simulink model "gm_hybrid_lht"  (R2019b)
settings: Solver=FixedStepDiscrete  StartTime=0.0  StopTime=inf  FixedStep=1/120e6  RelTol=1e-3
undefined symbols (not defined in the file or in its folder): bt, height, nTheta, width
libraries: hdlsllib x352, simulink x286, hdlmdlgenlib x7, dspsrcs4 x1
(part 9 of 12)

== system gm_hybrid_lht/Hybrid LHT/Hybrid LHT Accumulator/Accumulator with Switches/Accumulator_instance33/Block RAM/Simple Dual Port RAM Generator ==
  wr_data : Inport  OutDataTypeStr=fixdt(0, 36, 0)  PortDimensions=1  SampleTime=8.33333333333333e-09
  wr_addr : Inport  Port=2  OutDataTypeStr=fixdt(0, 11, 0)  PortDimensions=1  SampleTime=8.33333333333333e-09
  wr_en : Inport  Port=3  OutDataTypeStr=boolean  PortDimensions=1  SampleTime=8.33333333333333e-09
  rd_addr : Inport  Port=4  OutDataTypeStr=fixdt(0, 11, 0)  PortDimensions=1  SampleTime=8.33333333333333e-09
  and_0 : Logic  AllPortsSameDT=off  OutDataTypeStr=boolean
  and_1 : Logic  AllPortsSameDT=off  OutDataTypeStr=boolean
  bitwise_or : simulink/Logic and Bit Operations/Bitwise Operator  logicop=OR  UseBitMask=off  BitMask=bin2dec('11011001')  BitMaskRealWorld=Stored Integer
  constant_0 : Constant  Value=0  OutDataTypeStr=fixdt(0, 2, 0)  SampleTime=-1
  constant_1 : Constant  OutDataTypeStr=fixdt(0, 2, 0)  SampleTime=-1
  delay : Delay  DelayLength=1
  multiport_switch : MultiPortSwitch  DataPortOrder=Zero-based contiguous  Inputs=2  zeroidx=on
  rd_address : hdlsllib/Logic and Bit Operations/Bit Slice  lidx=9  ridx=0
      settings: SourceProductName=Simulink  SourceProductBaseCode=SL
  rd_address_hr : hdlsllib/Logic and Bit Operations/Bit Slice  lidx=8  ridx=0
      settings: SourceProductName=Simulink  SourceProductBaseCode=SL
  rd_bitslice : hdlsllib/Logic and Bit Operations/Bit Slice  lidx=10  ridx=10
      settings: SourceProductName=Simulink  SourceProductBaseCode=SL
  rd_cmp2const_0 : simulink/Logic and Bit Operations/Compare To Constant  relop===  const=0  OutDataTypeStr=boolean
  rd_cmp2const_1 : simulink/Logic and Bit Operations/Compare To Constant  relop===  const=1  OutDataTypeStr=boolean
  simple_ram_0 : hdlsllib/HDL RAMs/Simple Dual Port RAM  ram_size=10
      settings: SourceProductName=Simulink  SourceProductBaseCode=SL
  simple_ram_1 : hdlsllib/HDL RAMs/Simple Dual Port RAM  ram_size=9
      settings: SourceProductName=Simulink  SourceProductBaseCode=SL
  switch_0 : Switch  Threshold=1
  switch_1 : Switch  Threshold=1
  vector_concatenate : Concatenate
  wr_address : hdlsllib/Logic and Bit Operations/Bit Slice  lidx=9  ridx=0
      settings: SourceProductName=Simulink  SourceProductBaseCode=SL
  wr_address_hr : hdlsllib/Logic and Bit Operations/Bit Slice  lidx=8  ridx=0
      settings: SourceProductName=Simulink  SourceProductBaseCode=SL
  wr_bitslice : hdlsllib/Logic and Bit Operations/Bit Slice  lidx=10  ridx=10
      settings: SourceProductName=Simulink  SourceProductBaseCode=SL
  wr_cmp2const_0 : simulink/Logic and Bit Operations/Compare To Constant  relop===  const=0  OutDataTypeStr=boolean
  wr_cmp2const_1 : simulink/Logic and Bit Operations/Compare To Constant  relop===  const=1  OutDataTypeStr=boolean
  zero : Constant  Value=0  OutDataTypeStr=fixdt(0, 2, 0)  SampleTime=-1
  rd_data : Outport
  wires:
  rd_addr/1 -> rd_bitslice/1, rd_address_hr/1, rd_address/1
  wr_en/1 -> and_1/2, and_0/2
  wr_addr/1 -> wr_bitslice/1, wr_address_hr/1, wr_address/1
  wr_data/1 -> simple_ram_0/1, simple_ram_1/1
  and_0/1 -> simple_ram_0/3
  and_1/1 -> simple_ram_1/3
  bitwise_or/1 -> delay/1
  constant_0/1 -> switch_0/1
  constant_1/1 -> switch_1/1
  delay/1 -> multiport_switch/1
  multiport_switch/1 -> rd_data/1
  rd_address/1 -> simple_ram_0/4
  rd_address_hr/1 -> simple_ram_1/4
  rd_bitslice/1 -> rd_cmp2const_1/1, rd_cmp2const_0/1
  rd_cmp2const_0/1 -> switch_0/2
  rd_cmp2const_1/1 -> switch_1/2
  simple_ram_0/1 -> multiport_switch/2
  simple_ram_1/1 -> multiport_switch/3
  switch_0/1 -> vector_concatenate/1
  switch_1/1 -> vector_concatenate/2
  vector_concatenate/1 -> bitwise_or/1
  wr_address/1 -> simple_ram_0/2
  wr_address_hr/1 -> simple_ram_1/2
  wr_bitslice/1 -> wr_cmp2const_1/1, wr_cmp2const_0/1
  wr_cmp2const_0/1 -> and_0/1
  wr_cmp2const_1/1 -> and_1/1
  zero/1 -> switch_1/3, switch_0/3

== system gm_hybrid_lht/Hybrid LHT/Hybrid LHT Accumulator/Accumulator with Switches/Accumulator_instance34/Block RAM/Simple Dual Port RAM Generator ==
  wr_data : Inport  OutDataTypeStr=fixdt(0, 36, 0)  PortDimensions=1  SampleTime=8.33333333333333e-09
  wr_addr : Inport  Port=2  OutDataTypeStr=fixdt(0, 11, 0)  PortDimensions=1  SampleTime=8.33333333333333e-09
  wr_en : Inport  Port=3  OutDataTypeStr=boolean  PortDimensions=1  SampleTime=8.33333333333333e-09
  rd_addr : Inport  Port=4  OutDataTypeStr=fixdt(0, 11, 0)  PortDimensions=1  SampleTime=8.33333333333333e-09
  and_0 : Logic  AllPortsSameDT=off  OutDataTypeStr=boolean
  and_1 : Logic  AllPortsSameDT=off  OutDataTypeStr=boolean
  bitwise_or : simulink/Logic and Bit Operations/Bitwise Operator  logicop=OR  UseBitMask=off  BitMask=bin2dec('11011001')  BitMaskRealWorld=Stored Integer
  constant_0 : Constant  Value=0  OutDataTypeStr=fixdt(0, 2, 0)  SampleTime=-1
  constant_1 : Constant  OutDataTypeStr=fixdt(0, 2, 0)  SampleTime=-1
  delay : Delay  DelayLength=1
  multiport_switch : MultiPortSwitch  DataPortOrder=Zero-based contiguous  Inputs=2  zeroidx=on
  rd_address : hdlsllib/Logic and Bit Operations/Bit Slice  lidx=9  ridx=0
      settings: SourceProductName=Simulink  SourceProductBaseCode=SL
  rd_address_hr : hdlsllib/Logic and Bit Operations/Bit Slice  lidx=8  ridx=0
      settings: SourceProductName=Simulink  SourceProductBaseCode=SL
  rd_bitslice : hdlsllib/Logic and Bit Operations/Bit Slice  lidx=10  ridx=10
      settings: SourceProductName=Simulink  SourceProductBaseCode=SL
  rd_cmp2const_0 : simulink/Logic and Bit Operations/Compare To Constant  relop===  const=0  OutDataTypeStr=boolean
  rd_cmp2const_1 : simulink/Logic and Bit Operations/Compare To Constant  relop===  const=1  OutDataTypeStr=boolean
  simple_ram_0 : hdlsllib/HDL RAMs/Simple Dual Port RAM  ram_size=10
      settings: SourceProductName=Simulink  SourceProductBaseCode=SL
  simple_ram_1 : hdlsllib/HDL RAMs/Simple Dual Port RAM  ram_size=9
      settings: SourceProductName=Simulink  SourceProductBaseCode=SL
  switch_0 : Switch  Threshold=1
  switch_1 : Switch  Threshold=1
  vector_concatenate : Concatenate
  wr_address : hdlsllib/Logic and Bit Operations/Bit Slice  lidx=9  ridx=0
      settings: SourceProductName=Simulink  SourceProductBaseCode=SL
  wr_address_hr : hdlsllib/Logic and Bit Operations/Bit Slice  lidx=8  ridx=0
      settings: SourceProductName=Simulink  SourceProductBaseCode=SL
  wr_bitslice : hdlsllib/Logic and Bit Operations/Bit Slice  lidx=10  ridx=10
      settings: SourceProductName=Simulink  SourceProductBaseCode=SL
  wr_cmp2const_0 : simulink/Logic and Bit Operations/Compare To Constant  relop===  const=0  OutDataTypeStr=boolean
  wr_cmp2const_1 : simulink/Logic and Bit Operations/Compare To Constant  relop===  const=1  OutDataTypeStr=boolean
  zero : Constant  Value=0  OutDataTypeStr=fixdt(0, 2, 0)  SampleTime=-1
  rd_data : Outport
  wires:
  rd_addr/1 -> rd_bitslice/1, rd_address_hr/1, rd_address/1
  wr_en/1 -> and_1/2, and_0/2
  wr_addr/1 -> wr_bitslice/1, wr_address_hr/1, wr_address/1
  wr_data/1 -> simple_ram_0/1, simple_ram_1/1
  and_0/1 -> simple_ram_0/3
  and_1/1 -> simple_ram_1/3
  bitwise_or/1 -> delay/1
  constant_0/1 -> switch_0/1
  constant_1/1 -> switch_1/1
  delay/1 -> multiport_switch/1
  multiport_switch/1 -> rd_data/1
  rd_address/1 -> simple_ram_0/4
  rd_address_hr/1 -> simple_ram_1/4
  rd_bitslice/1 -> rd_cmp2const_1/1, rd_cmp2const_0/1
  rd_cmp2const_0/1 -> switch_0/2
  rd_cmp2const_1/1 -> switch_1/2
  simple_ram_0/1 -> multiport_switch/2
  simple_ram_1/1 -> multiport_switch/3
  switch_0/1 -> vector_concatenate/1
  switch_1/1 -> vector_concatenate/2
  vector_concatenate/1 -> bitwise_or/1
  wr_address/1 -> simple_ram_0/2
  wr_address_hr/1 -> simple_ram_1/2
  wr_bitslice/1 -> wr_cmp2const_1/1, wr_cmp2const_0/1
  wr_cmp2const_0/1 -> and_0/1
  wr_cmp2const_1/1 -> and_1/1
  zero/1 -> switch_1/3, switch_0/3

== system gm_hybrid_lht/Hybrid LHT/Hybrid LHT Accumulator/Accumulator with Switches/Accumulator_instance4/Block RAM/Simple Dual Port RAM Generator ==
  wr_data : Inport  OutDataTypeStr=fixdt(0, 36, 0)  PortDimensions=1  SampleTime=8.33333333333333e-09
  wr_addr : Inport  Port=2  OutDataTypeStr=fixdt(0, 11, 0)  PortDimensions=1  SampleTime=8.33333333333333e-09
  wr_en : Inport  Port=3  OutDataTypeStr=boolean  PortDimensions=1  SampleTime=8.33333333333333e-09
  rd_addr : Inport  Port=4  OutDataTypeStr=fixdt(0, 11, 0)  PortDimensions=1  SampleTime=8.33333333333333e-09
  and_0 : Logic  AllPortsSameDT=off  OutDataTypeStr=boolean
  and_1 : Logic  AllPortsSameDT=off  OutDataTypeStr=boolean
  bitwise_or : simulink/Logic and Bit Operations/Bitwise Operator  logicop=OR  UseBitMask=off  BitMask=bin2dec('11011001')  BitMaskRealWorld=Stored Integer
  constant_0 : Constant  Value=0  OutDataTypeStr=fixdt(0, 2, 0)  SampleTime=-1
  constant_1 : Constant  OutDataTypeStr=fixdt(0, 2, 0)  SampleTime=-1
  delay : Delay  DelayLength=1
  multiport_switch : MultiPortSwitch  DataPortOrder=Zero-based contiguous  Inputs=2  zeroidx=on
  rd_address : hdlsllib/Logic and Bit Operations/Bit Slice  lidx=9  ridx=0
      settings: SourceProductName=Simulink  SourceProductBaseCode=SL
  rd_address_hr : hdlsllib/Logic and Bit Operations/Bit Slice  lidx=8  ridx=0
      settings: SourceProductName=Simulink  SourceProductBaseCode=SL
  rd_bitslice : hdlsllib/Logic and Bit Operations/Bit Slice  lidx=10  ridx=10
      settings: SourceProductName=Simulink  SourceProductBaseCode=SL
  rd_cmp2const_0 : simulink/Logic and Bit Operations/Compare To Constant  relop===  const=0  OutDataTypeStr=boolean
  rd_cmp2const_1 : simulink/Logic and Bit Operations/Compare To Constant  relop===  const=1  OutDataTypeStr=boolean
  simple_ram_0 : hdlsllib/HDL RAMs/Simple Dual Port RAM  ram_size=10
      settings: SourceProductName=Simulink  SourceProductBaseCode=SL
  simple_ram_1 : hdlsllib/HDL RAMs/Simple Dual Port RAM  ram_size=9
      settings: SourceProductName=Simulink  SourceProductBaseCode=SL
  switch_0 : Switch  Threshold=1
  switch_1 : Switch  Threshold=1
  vector_concatenate : Concatenate
  wr_address : hdlsllib/Logic and Bit Operations/Bit Slice  lidx=9  ridx=0
      settings: SourceProductName=Simulink  SourceProductBaseCode=SL
  wr_address_hr : hdlsllib/Logic and Bit Operations/Bit Slice  lidx=8  ridx=0
      settings: SourceProductName=Simulink  SourceProductBaseCode=SL
  wr_bitslice : hdlsllib/Logic and Bit Operations/Bit Slice  lidx=10  ridx=10
      settings: SourceProductName=Simulink  SourceProductBaseCode=SL
  wr_cmp2const_0 : simulink/Logic and Bit Operations/Compare To Constant  relop===  const=0  OutDataTypeStr=boolean
  wr_cmp2const_1 : simulink/Logic and Bit Operations/Compare To Constant  relop===  const=1  OutDataTypeStr=boolean
  zero : Constant  Value=0  OutDataTypeStr=fixdt(0, 2, 0)  SampleTime=-1
  rd_data : Outport
  wires:
  rd_addr/1 -> rd_bitslice/1, rd_address_hr/1, rd_address/1
  wr_en/1 -> and_1/2, and_0/2
  wr_addr/1 -> wr_bitslice/1, wr_address_hr/1, wr_address/1
  wr_data/1 -> simple_ram_0/1, simple_ram_1/1
  and_0/1 -> simple_ram_0/3
  and_1/1 -> simple_ram_1/3
  bitwise_or/1 -> delay/1
  constant_0/1 -> switch_0/1
  constant_1/1 -> switch_1/1
  delay/1 -> multiport_switch/1
  multiport_switch/1 -> rd_data/1
  rd_address/1 -> simple_ram_0/4
  rd_address_hr/1 -> simple_ram_1/4
  rd_bitslice/1 -> rd_cmp2const_1/1, rd_cmp2const_0/1
  rd_cmp2const_0/1 -> switch_0/2
  rd_cmp2const_1/1 -> switch_1/2
  simple_ram_0/1 -> multiport_switch/2
  simple_ram_1/1 -> multiport_switch/3
  switch_0/1 -> vector_concatenate/1
  switch_1/1 -> vector_concatenate/2
  vector_concatenate/1 -> bitwise_or/1
  wr_address/1 -> simple_ram_0/2
  wr_address_hr/1 -> simple_ram_1/2
  wr_bitslice/1 -> wr_cmp2const_1/1, wr_cmp2const_0/1
  wr_cmp2const_0/1 -> and_0/1
  wr_cmp2const_1/1 -> and_1/1
  zero/1 -> switch_1/3, switch_0/3

== system gm_hybrid_lht/Hybrid LHT/Hybrid LHT Accumulator/Accumulator with Switches/Accumulator_instance5/Block RAM/Simple Dual Port RAM Generator ==
  wr_data : Inport  OutDataTypeStr=fixdt(0, 36, 0)  PortDimensions=1  SampleTime=8.33333333333333e-09
  wr_addr : Inport  Port=2  OutDataTypeStr=fixdt(0, 11, 0)  PortDimensions=1  SampleTime=8.33333333333333e-09
  wr_en : Inport  Port=3  OutDataTypeStr=boolean  PortDimensions=1  SampleTime=8.33333333333333e-09
  rd_addr : Inport  Port=4  OutDataTypeStr=fixdt(0, 11, 0)  PortDimensions=1  SampleTime=8.33333333333333e-09
  and_0 : Logic  AllPortsSameDT=off  OutDataTypeStr=boolean
  and_1 : Logic  AllPortsSameDT=off  OutDataTypeStr=boolean
  bitwise_or : simulink/Logic and Bit Operations/Bitwise Operator  logicop=OR  UseBitMask=off  BitMask=bin2dec('11011001')  BitMaskRealWorld=Stored Integer
  constant_0 : Constant  Value=0  OutDataTypeStr=fixdt(0, 2, 0)  SampleTime=-1
  constant_1 : Constant  OutDataTypeStr=fixdt(0, 2, 0)  SampleTime=-1
  delay : Delay  DelayLength=1
  multiport_switch : MultiPortSwitch  DataPortOrder=Zero-based contiguous  Inputs=2  zeroidx=on
  rd_address : hdlsllib/Logic and Bit Operations/Bit Slice  lidx=9  ridx=0
      settings: SourceProductName=Simulink  SourceProductBaseCode=SL
  rd_address_hr : hdlsllib/Logic and Bit Operations/Bit Slice  lidx=8  ridx=0
      settings: SourceProductName=Simulink  SourceProductBaseCode=SL
  rd_bitslice : hdlsllib/Logic and Bit Operations/Bit Slice  lidx=10  ridx=10
      settings: SourceProductName=Simulink  SourceProductBaseCode=SL
  rd_cmp2const_0 : simulink/Logic and Bit Operations/Compare To Constant  relop===  const=0  OutDataTypeStr=boolean
  rd_cmp2const_1 : simulink/Logic and Bit Operations/Compare To Constant  relop===  const=1  OutDataTypeStr=boolean
  simple_ram_0 : hdlsllib/HDL RAMs/Simple Dual Port RAM  ram_size=10
      settings: SourceProductName=Simulink  SourceProductBaseCode=SL
  simple_ram_1 : hdlsllib/HDL RAMs/Simple Dual Port RAM  ram_size=9
      settings: SourceProductName=Simulink  SourceProductBaseCode=SL
  switch_0 : Switch  Threshold=1
  switch_1 : Switch  Threshold=1
  vector_concatenate : Concatenate
  wr_address : hdlsllib/Logic and Bit Operations/Bit Slice  lidx=9  ridx=0
      settings: SourceProductName=Simulink  SourceProductBaseCode=SL
  wr_address_hr : hdlsllib/Logic and Bit Operations/Bit Slice  lidx=8  ridx=0
      settings: SourceProductName=Simulink  SourceProductBaseCode=SL
  wr_bitslice : hdlsllib/Logic and Bit Operations/Bit Slice  lidx=10  ridx=10
      settings: SourceProductName=Simulink  SourceProductBaseCode=SL
  wr_cmp2const_0 : simulink/Logic and Bit Operations/Compare To Constant  relop===  const=0  OutDataTypeStr=boolean
  wr_cmp2const_1 : simulink/Logic and Bit Operations/Compare To Constant  relop===  const=1  OutDataTypeStr=boolean
  zero : Constant  Value=0  OutDataTypeStr=fixdt(0, 2, 0)  SampleTime=-1
  rd_data : Outport
  wires:
  rd_addr/1 -> rd_bitslice/1, rd_address_hr/1, rd_address/1
  wr_en/1 -> and_1/2, and_0/2
  wr_addr/1 -> wr_bitslice/1, wr_address_hr/1, wr_address/1
  wr_data/1 -> simple_ram_0/1, simple_ram_1/1
  and_0/1 -> simple_ram_0/3
  and_1/1 -> simple_ram_1/3
  bitwise_or/1 -> delay/1
  constant_0/1 -> switch_0/1
  constant_1/1 -> switch_1/1
  delay/1 -> multiport_switch/1
  multiport_switch/1 -> rd_data/1
  rd_address/1 -> simple_ram_0/4
  rd_address_hr/1 -> simple_ram_1/4
  rd_bitslice/1 -> rd_cmp2const_1/1, rd_cmp2const_0/1
  rd_cmp2const_0/1 -> switch_0/2
  rd_cmp2const_1/1 -> switch_1/2
  simple_ram_0/1 -> multiport_switch/2
  simple_ram_1/1 -> multiport_switch/3
  switch_0/1 -> vector_concatenate/1
  switch_1/1 -> vector_concatenate/2
  vector_concatenate/1 -> bitwise_or/1
  wr_address/1 -> simple_ram_0/2
  wr_address_hr/1 -> simple_ram_1/2
  wr_bitslice/1 -> wr_cmp2const_1/1, wr_cmp2const_0/1
  wr_cmp2const_0/1 -> and_0/1
  wr_cmp2const_1/1 -> and_1/1
  zero/1 -> switch_1/3, switch_0/3

== system gm_hybrid_lht/Hybrid LHT/Hybrid LHT Accumulator/Accumulator with Switches/Accumulator_instance6/Block RAM/Simple Dual Port RAM Generator ==
  wr_data : Inport  OutDataTypeStr=fixdt(0, 36, 0)  PortDimensions=1  SampleTime=8.33333333333333e-09
  wr_addr : Inport  Port=2  OutDataTypeStr=fixdt(0, 11, 0)  PortDimensions=1  SampleTime=8.33333333333333e-09
  wr_en : Inport  Port=3  OutDataTypeStr=boolean  PortDimensions=1  SampleTime=8.33333333333333e-09
  rd_addr : Inport  Port=4  OutDataTypeStr=fixdt(0, 11, 0)  PortDimensions=1  SampleTime=8.33333333333333e-09
  and_0 : Logic  AllPortsSameDT=off  OutDataTypeStr=boolean
  and_1 : Logic  AllPortsSameDT=off  OutDataTypeStr=boolean
  bitwise_or : simulink/Logic and Bit Operations/Bitwise Operator  logicop=OR  UseBitMask=off  BitMask=bin2dec('11011001')  BitMaskRealWorld=Stored Integer
  constant_0 : Constant  Value=0  OutDataTypeStr=fixdt(0, 2, 0)  SampleTime=-1
  constant_1 : Constant  OutDataTypeStr=fixdt(0, 2, 0)  SampleTime=-1
  delay : Delay  DelayLength=1
  multiport_switch : MultiPortSwitch  DataPortOrder=Zero-based contiguous  Inputs=2  zeroidx=on
  rd_address : hdlsllib/Logic and Bit Operations/Bit Slice  lidx=9  ridx=0
      settings: SourceProductName=Simulink  SourceProductBaseCode=SL
  rd_address_hr : hdlsllib/Logic and Bit Operations/Bit Slice  lidx=8  ridx=0
      settings: SourceProductName=Simulink  SourceProductBaseCode=SL
  rd_bitslice : hdlsllib/Logic and Bit Operations/Bit Slice  lidx=10  ridx=10
      settings: SourceProductName=Simulink  SourceProductBaseCode=SL
  rd_cmp2const_0 : simulink/Logic and Bit Operations/Compare To Constant  relop===  const=0  OutDataTypeStr=boolean
  rd_cmp2const_1 : simulink/Logic and Bit Operations/Compare To Constant  relop===  const=1  OutDataTypeStr=boolean
  simple_ram_0 : hdlsllib/HDL RAMs/Simple Dual Port RAM  ram_size=10
      settings: SourceProductName=Simulink  SourceProductBaseCode=SL
  simple_ram_1 : hdlsllib/HDL RAMs/Simple Dual Port RAM  ram_size=9
      settings: SourceProductName=Simulink  SourceProductBaseCode=SL
  switch_0 : Switch  Threshold=1
  switch_1 : Switch  Threshold=1
  vector_concatenate : Concatenate
  wr_address : hdlsllib/Logic and Bit Operations/Bit Slice  lidx=9  ridx=0
      settings: SourceProductName=Simulink  SourceProductBaseCode=SL
  wr_address_hr : hdlsllib/Logic and Bit Operations/Bit Slice  lidx=8  ridx=0
      settings: SourceProductName=Simulink  SourceProductBaseCode=SL
  wr_bitslice : hdlsllib/Logic and Bit Operations/Bit Slice  lidx=10  ridx=10
      settings: SourceProductName=Simulink  SourceProductBaseCode=SL
  wr_cmp2const_0 : simulink/Logic and Bit Operations/Compare To Constant  relop===  const=0  OutDataTypeStr=boolean
  wr_cmp2const_1 : simulink/Logic and Bit Operations/Compare To Constant  relop===  const=1  OutDataTypeStr=boolean
  zero : Constant  Value=0  OutDataTypeStr=fixdt(0, 2, 0)  SampleTime=-1
  rd_data : Outport
  wires:
  rd_addr/1 -> rd_bitslice/1, rd_address_hr/1, rd_address/1
  wr_en/1 -> and_1/2, and_0/2
  wr_addr/1 -> wr_bitslice/1, wr_address_hr/1, wr_address/1
  wr_data/1 -> simple_ram_0/1, simple_ram_1/1
  and_0/1 -> simple_ram_0/3
  and_1/1 -> simple_ram_1/3
  bitwise_or/1 -> delay/1
  constant_0/1 -> switch_0/1
  constant_1/1 -> switch_1/1
  delay/1 -> multiport_switch/1
  multiport_switch/1 -> rd_data/1
  rd_address/1 -> simple_ram_0/4
  rd_address_hr/1 -> simple_ram_1/4
  rd_bitslice/1 -> rd_cmp2const_1/1, rd_cmp2const_0/1
  rd_cmp2const_0/1 -> switch_0/2
  rd_cmp2const_1/1 -> switch_1/2
  simple_ram_0/1 -> multiport_switch/2
  simple_ram_1/1 -> multiport_switch/3
  switch_0/1 -> vector_concatenate/1
  switch_1/1 -> vector_concatenate/2
  vector_concatenate/1 -> bitwise_or/1
  wr_address/1 -> simple_ram_0/2
  wr_address_hr/1 -> simple_ram_1/2
  wr_bitslice/1 -> wr_cmp2const_1/1, wr_cmp2const_0/1
  wr_cmp2const_0/1 -> and_0/1
  wr_cmp2const_1/1 -> and_1/1
  zero/1 -> switch_1/3, switch_0/3

== system gm_hybrid_lht/Hybrid LHT/Hybrid LHT Accumulator/Accumulator with Switches/Accumulator_instance7/Block RAM/Simple Dual Port RAM Generator ==
  wr_data : Inport  OutDataTypeStr=fixdt(0, 36, 0)  PortDimensions=1  SampleTime=8.33333333333333e-09
  wr_addr : Inport  Port=2  OutDataTypeStr=fixdt(0, 11, 0)  PortDimensions=1  SampleTime=8.33333333333333e-09
  wr_en : Inport  Port=3  OutDataTypeStr=boolean  PortDimensions=1  SampleTime=8.33333333333333e-09
  rd_addr : Inport  Port=4  OutDataTypeStr=fixdt(0, 11, 0)  PortDimensions=1  SampleTime=8.33333333333333e-09
  and_0 : Logic  AllPortsSameDT=off  OutDataTypeStr=boolean
  and_1 : Logic  AllPortsSameDT=off  OutDataTypeStr=boolean
  bitwise_or : simulink/Logic and Bit Operations/Bitwise Operator  logicop=OR  UseBitMask=off  BitMask=bin2dec('11011001')  BitMaskRealWorld=Stored Integer
  constant_0 : Constant  Value=0  OutDataTypeStr=fixdt(0, 2, 0)  SampleTime=-1
  constant_1 : Constant  OutDataTypeStr=fixdt(0, 2, 0)  SampleTime=-1
  delay : Delay  DelayLength=1
  multiport_switch : MultiPortSwitch  DataPortOrder=Zero-based contiguous  Inputs=2  zeroidx=on
  rd_address : hdlsllib/Logic and Bit Operations/Bit Slice  lidx=9  ridx=0
      settings: SourceProductName=Simulink  SourceProductBaseCode=SL
  rd_address_hr : hdlsllib/Logic and Bit Operations/Bit Slice  lidx=8  ridx=0
      settings: SourceProductName=Simulink  SourceProductBaseCode=SL
  rd_bitslice : hdlsllib/Logic and Bit Operations/Bit Slice  lidx=10  ridx=10
      settings: SourceProductName=Simulink  SourceProductBaseCode=SL
  rd_cmp2const_0 : simulink/Logic and Bit Operations/Compare To Constant  relop===  const=0  OutDataTypeStr=boolean
  rd_cmp2const_1 : simulink/Logic and Bit Operations/Compare To Constant  relop===  const=1  OutDataTypeStr=boolean
  simple_ram_0 : hdlsllib/HDL RAMs/Simple Dual Port RAM  ram_size=10
      settings: SourceProductName=Simulink  SourceProductBaseCode=SL
  simple_ram_1 : hdlsllib/HDL RAMs/Simple Dual Port RAM  ram_size=9
      settings: SourceProductName=Simulink  SourceProductBaseCode=SL
  switch_0 : Switch  Threshold=1
  switch_1 : Switch  Threshold=1
  vector_concatenate : Concatenate
  wr_address : hdlsllib/Logic and Bit Operations/Bit Slice  lidx=9  ridx=0
      settings: SourceProductName=Simulink  SourceProductBaseCode=SL
  wr_address_hr : hdlsllib/Logic and Bit Operations/Bit Slice  lidx=8  ridx=0
      settings: SourceProductName=Simulink  SourceProductBaseCode=SL
  wr_bitslice : hdlsllib/Logic and Bit Operations/Bit Slice  lidx=10  ridx=10
      settings: SourceProductName=Simulink  SourceProductBaseCode=SL
  wr_cmp2const_0 : simulink/Logic and Bit Operations/Compare To Constant  relop===  const=0  OutDataTypeStr=boolean
  wr_cmp2const_1 : simulink/Logic and Bit Operations/Compare To Constant  relop===  const=1  OutDataTypeStr=boolean
  zero : Constant  Value=0  OutDataTypeStr=fixdt(0, 2, 0)  SampleTime=-1
  rd_data : Outport
  wires:
  rd_addr/1 -> rd_bitslice/1, rd_address_hr/1, rd_address/1
  wr_en/1 -> and_1/2, and_0/2
  wr_addr/1 -> wr_bitslice/1, wr_address_hr/1, wr_address/1
  wr_data/1 -> simple_ram_0/1, simple_ram_1/1
  and_0/1 -> simple_ram_0/3
  and_1/1 -> simple_ram_1/3
  bitwise_or/1 -> delay/1
  constant_0/1 -> switch_0/1
  constant_1/1 -> switch_1/1
  delay/1 -> multiport_switch/1
  multiport_switch/1 -> rd_data/1
  rd_address/1 -> simple_ram_0/4
  rd_address_hr/1 -> simple_ram_1/4
  rd_bitslice/1 -> rd_cmp2const_1/1, rd_cmp2const_0/1
  rd_cmp2const_0/1 -> switch_0/2
  rd_cmp2const_1/1 -> switch_1/2
  simple_ram_0/1 -> multiport_switch/2
  simple_ram_1/1 -> multiport_switch/3
  switch_0/1 -> vector_concatenate/1
  switch_1/1 -> vector_concatenate/2
  vector_concatenate/1 -> bitwise_or/1
  wr_address/1 -> simple_ram_0/2
  wr_address_hr/1 -> simple_ram_1/2
  wr_bitslice/1 -> wr_cmp2const_1/1, wr_cmp2const_0/1
  wr_cmp2const_0/1 -> and_0/1
  wr_cmp2const_1/1 -> and_1/1
  zero/1 -> switch_1/3, switch_0/3

== system gm_hybrid_lht/Hybrid LHT/Hybrid LHT Accumulator/Accumulator with Switches/Accumulator_instance8/Block RAM/Simple Dual Port RAM Generator ==
  wr_data : Inport  OutDataTypeStr=fixdt(0, 36, 0)  PortDimensions=1  SampleTime=8.33333333333333e-09
  wr_addr : Inport  Port=2  OutDataTypeStr=fixdt(0, 11, 0)  PortDimensions=1  SampleTime=8.33333333333333e-09
  wr_en : Inport  Port=3  OutDataTypeStr=boolean  PortDimensions=1  SampleTime=8.33333333333333e-09
  rd_addr : Inport  Port=4  OutDataTypeStr=fixdt(0, 11, 0)  PortDimensions=1  SampleTime=8.33333333333333e-09
  and_0 : Logic  AllPortsSameDT=off  OutDataTypeStr=boolean
  and_1 : Logic  AllPortsSameDT=off  OutDataTypeStr=boolean
  bitwise_or : simulink/Logic and Bit Operations/Bitwise Operator  logicop=OR  UseBitMask=off  BitMask=bin2dec('11011001')  BitMaskRealWorld=Stored Integer
  constant_0 : Constant  Value=0  OutDataTypeStr=fixdt(0, 2, 0)  SampleTime=-1
  constant_1 : Constant  OutDataTypeStr=fixdt(0, 2, 0)  SampleTime=-1
  delay : Delay  DelayLength=1
  multiport_switch : MultiPortSwitch  DataPortOrder=Zero-based contiguous  Inputs=2  zeroidx=on
  rd_address : hdlsllib/Logic and Bit Operations/Bit Slice  lidx=9  ridx=0
      settings: SourceProductName=Simulink  SourceProductBaseCode=SL
  rd_address_hr : hdlsllib/Logic and Bit Operations/Bit Slice  lidx=8  ridx=0
      settings: SourceProductName=Simulink  SourceProductBaseCode=SL
  rd_bitslice : hdlsllib/Logic and Bit Operations/Bit Slice  lidx=10  ridx=10
      settings: SourceProductName=Simulink  SourceProductBaseCode=SL
  rd_cmp2const_0 : simulink/Logic and Bit Operations/Compare To Constant  relop===  const=0  OutDataTypeStr=boolean
  rd_cmp2const_1 : simulink/Logic and Bit Operations/Compare To Constant  relop===  const=1  OutDataTypeStr=boolean
  simple_ram_0 : hdlsllib/HDL RAMs/Simple Dual Port RAM  ram_size=10
      settings: SourceProductName=Simulink  SourceProductBaseCode=SL
  simple_ram_1 : hdlsllib/HDL RAMs/Simple Dual Port RAM  ram_size=9
      settings: SourceProductName=Simulink  SourceProductBaseCode=SL
  switch_0 : Switch  Threshold=1
  switch_1 : Switch  Threshold=1
  vector_concatenate : Concatenate
  wr_address : hdlsllib/Logic and Bit Operations/Bit Slice  lidx=9  ridx=0
      settings: SourceProductName=Simulink  SourceProductBaseCode=SL
  wr_address_hr : hdlsllib/Logic and Bit Operations/Bit Slice  lidx=8  ridx=0
      settings: SourceProductName=Simulink  SourceProductBaseCode=SL
  wr_bitslice : hdlsllib/Logic and Bit Operations/Bit Slice  lidx=10  ridx=10
      settings: SourceProductName=Simulink  SourceProductBaseCode=SL
  wr_cmp2const_0 : simulink/Logic and Bit Operations/Compare To Constant  relop===  const=0  OutDataTypeStr=boolean
  wr_cmp2const_1 : simulink/Logic and Bit Operations/Compare To Constant  relop===  const=1  OutDataTypeStr=boolean
  zero : Constant  Value=0  OutDataTypeStr=fixdt(0, 2, 0)  SampleTime=-1
  rd_data : Outport
  wires:
  rd_addr/1 -> rd_bitslice/1, rd_address_hr/1, rd_address/1
  wr_en/1 -> and_1/2, and_0/2
  wr_addr/1 -> wr_bitslice/1, wr_address_hr/1, wr_address/1
  wr_data/1 -> simple_ram_0/1, simple_ram_1/1
  and_0/1 -> simple_ram_0/3
  and_1/1 -> simple_ram_1/3
  bitwise_or/1 -> delay/1
  constant_0/1 -> switch_0/1
  constant_1/1 -> switch_1/1
  delay/1 -> multiport_switch/1
  multiport_switch/1 -> rd_data/1
  rd_address/1 -> simple_ram_0/4
  rd_address_hr/1 -> simple_ram_1/4
  rd_bitslice/1 -> rd_cmp2const_1/1, rd_cmp2const_0/1
  rd_cmp2const_0/1 -> switch_0/2
  rd_cmp2const_1/1 -> switch_1/2
  simple_ram_0/1 -> multiport_switch/2
  simple_ram_1/1 -> multiport_switch/3
  switch_0/1 -> vector_concatenate/1
  switch_1/1 -> vector_concatenate/2
  vector_concatenate/1 -> bitwise_or/1
  wr_address/1 -> simple_ram_0/2
  wr_address_hr/1 -> simple_ram_1/2
  wr_bitslice/1 -> wr_cmp2const_1/1, wr_cmp2const_0/1
  wr_cmp2const_0/1 -> and_0/1
  wr_cmp2const_1/1 -> and_1/1
  zero/1 -> switch_1/3, switch_0/3

== system gm_hybrid_lht/Hybrid LHT/Hybrid LHT Accumulator/Accumulator with Switches/Accumulator_instance9/Block RAM/Simple Dual Port RAM Generator ==
  wr_data : Inport  OutDataTypeStr=fixdt(0, 36, 0)  PortDimensions=1  SampleTime=8.33333333333333e-09
  wr_addr : Inport  Port=2  OutDataTypeStr=fixdt(0, 11, 0)  PortDimensions=1  SampleTime=8.33333333333333e-09
  wr_en : Inport  Port=3  OutDataTypeStr=boolean  PortDimensions=1  SampleTime=8.33333333333333e-09
  rd_addr : Inport  Port=4  OutDataTypeStr=fixdt(0, 11, 0)  PortDimensions=1  SampleTime=8.33333333333333e-09
  and_0 : Logic  AllPortsSameDT=off  OutDataTypeStr=boolean
  and_1 : Logic  AllPortsSameDT=off  OutDataTypeStr=boolean
  bitwise_or : simulink/Logic and Bit Operations/Bitwise Operator  logicop=OR  UseBitMask=off  BitMask=bin2dec('11011001')  BitMaskRealWorld=Stored Integer
  constant_0 : Constant  Value=0  OutDataTypeStr=fixdt(0, 2, 0)  SampleTime=-1
  constant_1 : Constant  OutDataTypeStr=fixdt(0, 2, 0)  SampleTime=-1
  delay : Delay  DelayLength=1
  multiport_switch : MultiPortSwitch  DataPortOrder=Zero-based contiguous  Inputs=2  zeroidx=on
  rd_address : hdlsllib/Logic and Bit Operations/Bit Slice  lidx=9  ridx=0
      settings: SourceProductName=Simulink  SourceProductBaseCode=SL
  rd_address_hr : hdlsllib/Logic and Bit Operations/Bit Slice  lidx=8  ridx=0
      settings: SourceProductName=Simulink  SourceProductBaseCode=SL
  rd_bitslice : hdlsllib/Logic and Bit Operations/Bit Slice  lidx=10  ridx=10
      settings: SourceProductName=Simulink  SourceProductBaseCode=SL
  rd_cmp2const_0 : simulink/Logic and Bit Operations/Compare To Constant  relop===  const=0  OutDataTypeStr=boolean
  rd_cmp2const_1 : simulink/Logic and Bit Operations/Compare To Constant  relop===  const=1  OutDataTypeStr=boolean
  simple_ram_0 : hdlsllib/HDL RAMs/Simple Dual Port RAM  ram_size=10
      settings: SourceProductName=Simulink  SourceProductBaseCode=SL
  simple_ram_1 : hdlsllib/HDL RAMs/Simple Dual Port RAM  ram_size=9
      settings: SourceProductName=Simulink  SourceProductBaseCode=SL
  switch_0 : Switch  Threshold=1
  switch_1 : Switch  Threshold=1
  vector_concatenate : Concatenate
  wr_address : hdlsllib/Logic and Bit Operations/Bit Slice  lidx=9  ridx=0
      settings: SourceProductName=Simulink  SourceProductBaseCode=SL
  wr_address_hr : hdlsllib/Logic and Bit Operations/Bit Slice  lidx=8  ridx=0
      settings: SourceProductName=Simulink  SourceProductBaseCode=SL
  wr_bitslice : hdlsllib/Logic and Bit Operations/Bit Slice  lidx=10  ridx=10
      settings: SourceProductName=Simulink  SourceProductBaseCode=SL
  wr_cmp2const_0 : simulink/Logic and Bit Operations/Compare To Constant  relop===  const=0  OutDataTypeStr=boolean
  wr_cmp2const_1 : simulink/Logic and Bit Operations/Compare To Constant  relop===  const=1  OutDataTypeStr=boolean
  zero : Constant  Value=0  OutDataTypeStr=fixdt(0, 2, 0)  SampleTime=-1
  rd_data : Outport
  wires:
  rd_addr/1 -> rd_bitslice/1, rd_address_hr/1, rd_address/1
  wr_en/1 -> and_1/2, and_0/2
  wr_addr/1 -> wr_bitslice/1, wr_address_hr/1, wr_address/1
  wr_data/1 -> simple_ram_0/1, simple_ram_1/1
  and_0/1 -> simple_ram_0/3
  and_1/1 -> simple_ram_1/3
  bitwise_or/1 -> delay/1
  constant_0/1 -> switch_0/1
  constant_1/1 -> switch_1/1
  delay/1 -> multiport_switch/1
  multiport_switch/1 -> rd_data/1
  rd_address/1 -> simple_ram_0/4
  rd_address_hr/1 -> simple_ram_1/4
  rd_bitslice/1 -> rd_cmp2const_1/1, rd_cmp2const_0/1
  rd_cmp2const_0/1 -> switch_0/2
  rd_cmp2const_1/1 -> switch_1/2
  simple_ram_0/1 -> multiport_switch/2
  simple_ram_1/1 -> multiport_switch/3
  switch_0/1 -> vector_concatenate/1
  switch_1/1 -> vector_concatenate/2
  vector_concatenate/1 -> bitwise_or/1
  wr_address/1 -> simple_ram_0/2
  wr_address_hr/1 -> simple_ram_1/2
  wr_bitslice/1 -> wr_cmp2const_1/1, wr_cmp2const_0/1
  wr_cmp2const_0/1 -> and_0/1
  wr_cmp2const_1/1 -> and_1/1
  zero/1 -> switch_1/3, switch_0/3
